simulink model "PIDPositionerF141"  (Simulink 9.1)
settings: Solver=ode4  StartTime=0.0  StopTime=3  RelTol=1e-3  EnableMultiTasking=on
StopFcn:
  | %extract data from structure and plot vs time
  | %Birdsong 10/20/06
  | %This file is copied into the PIDPositioner.mdl Stop callback function
  | %at file/model properites/Callbacks/StopFcn
  | %extract vectors from structure data
  | 
  | %first extract vector data from structure data
  | pid_out=expdata.signals(1).values;
  | des_pos=expdata.signals(2).values(:,1);
  | meas_pos=expdata.signals(2).values(:,2);
  | t=expdata.time;
  | 
  | %plot data in a new figure
  | figure(1);subplot(211)
  | plot(t,pid_out);grid;
  | %axis([0,5,-12,12]);
  | xlabel('Time (sec)');
  | ylabel('PID Controller Ouput (volts)');
  | kp=get_param(strcat(gcs,'/PID Controller'), 'P'); %must match mdl file name exactly
  | ki=get_param(strcat(gcs,'/PID Controller'), 'I');
  | kd=get_param(strcat(gcs,'/PID Controller'), 'D');
  | plot_title=['Closed-Loop PID Controller Sysetm Response Kp=' num2str(kp) ', Ki=' num2str(ki) ', Kd=' num2str(kd)];
  | title(plot_title);
  | 
  | subplot(212);
  | plot(t,des_pos,'--',t,meas_pos,'-');grid;
  | xlabel('Time (sec)');
  | ylabel('Displacement (inches)');
  | legend('desired','measured');
  | %maxlim=1.1*max(max(meas_pos(2000:5000)),max(des_pos(2000:5000)));
  | %minlim=1.1*min(min(meas_pos(2000:5000)),min(des_pos(2000:5000)));
  | %axis([0,5,minlim,maxlim]); %adjust scale account for large offset from any initial drift
values from neighbouring files (symbols this model uses):
  expdata =     [PD10_0.01workspace.mat]    (also in PD42.5_0.1workspace.mat; PID47.5_12_0.15workspace.mat; POnly82workspace.mat; rampP10workspace.mat)
undefined symbols (not defined in the file or in its folder): MIO, National_Instruments, PCI
libraries: sldrtlib x2, simulink_need_slupdate x1, simulink x1
settings Model: Creator=Houska  LastModifiedBy=melab2  SimulationMode=external  ExtModeTrigDuration=10000
settings DataIOCC: LimitDataPoints=on  SignalLoggingSaveFormat=ModelDataLogs  SaveOutput=off  SaveTime=off  SignalLoggingName=logsOut
settings OptimizationCC: ExpressionDepthLimit=2147483647  InitFltsAndDblsToZero=on  LifeSpan=auto
settings DebuggingCC: SaveWithParameterizedLinksMsg=none  SignalResolutionControl=TryResolveAllWithWarning  MultiTaskDSMMsg=warning  MultiTaskCondExecSysMsg=none  FcnCallInpInsideContextMsg=warning  StateNameClashWarn=warning
settings HardwareCC: ProdBitPerPointer=64  ProdBitPerSizeT=64  ProdBitPerPtrDiffT=64  ProdLargestAtomicFloat=Float  ProdIntDivRoundTo=Zero  ProdEndianess=LittleEndian  ProdWordSize=64  ProdHWDeviceType=Intel->x86-64 (Windows64)
settings RTWCC: SystemTargetFile=sldrt.tlc  TemplateMakefile=sldrt.tmf  Description=Simulink Desktop Real-Time  RTWCompilerOptimization=on
settings CodeAppCC: MaxIdLength=95
settings SimulinkDesktopRealTimeCC: TargetPreCompLibLocation=C:\Program Files\MATLAB\R2018a\toolbox\sldrt\lib\win64  TargetLangStandard=C89/C90 (ANSI)  ModelReferenceCompliant=off  CompOptLevelCompliant=off  SupportVariableSizeSignals=off
settings ConfigComp: CovSFcnEnable=off

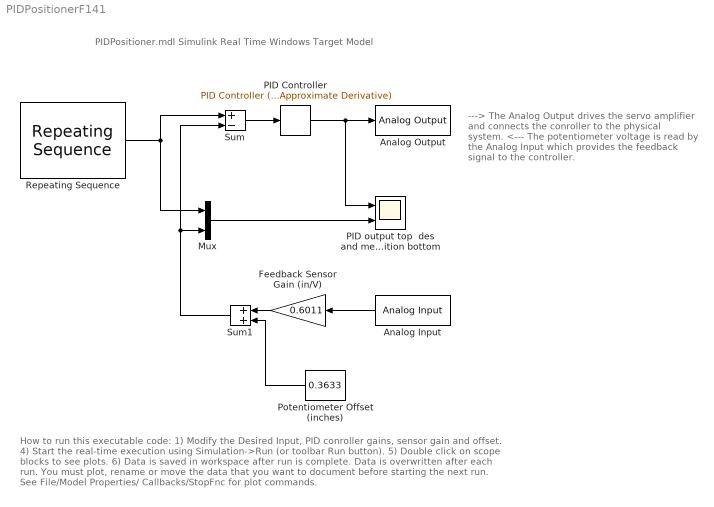
== system PIDPositionerF141 ==
  note: How to run this executable code:
      |
      | 1) Modify the Desired Input, PID conroller gains, sensor gain and offset.
      |
      | 4) Start the real-time execution using Simulation->Run (or toolbar Run button).
      |
      | 5) Double click on scope blocks to see plots.
      |
      | 6) Data is saved in workspace after run is complete.  Data is overwritten after each run.  You must plot,
      | rename or move the data that you want to document before starting the next run.  See File/Model Properties/
      | Callbacks/StopFnc for plot commands.
  note: ---> The Analog Output drives
      | the servo amplifier and
      | connects the conroller to
      | the physical system.
      |
      |
      |
      |
      |
      |
      |
      |
      | <--- The potentiometer voltage
      | is read by the Analog Input
      | which provides the feedback
      | signal to the controller.
  note: PIDPositioner.mdl
      | Simulink Real Time Windows Target Model
  Analog Input : sldrtlib/Analog Input  SampleTime=1e-3  MaxMissedTicks=10  ShowMissedTicks=off  YieldWhenWaiting=off  DrvName=National_Instruments/PCI-MIO-16E-4  DrvAddress=4294967295  DrvOptions=[0 0 0 0 0]  Channels=2  RangeMode=1  VoltRange=1  DataType=1
      settings: AttributesFormatString=National Instruments\nPCI-MIO-16E-4 [auto]  SourceProductName=Simulink Desktop Real-Time
  Analog Output : sldrtlib/Analog Output  SampleTime=1e-3  MaxMissedTicks=10  ShowMissedTicks=off  YieldWhenWaiting=off  DrvName=National_Instruments/PCI-MIO-16E-4  DrvAddress=4294967295  DrvOptions=[0 0 0 0 0]  Channels=1  RangeMode=1  VoltRange=1  InitialValue=0  FinalValue=0
      settings: AttributesFormatString=National Instruments\nPCI-MIO-16E-4 [auto]  SourceProductName=Simulink Desktop Real-Time
  Feedback Sensor Gain (in/V) : Gain  Gain=0.6011
  Mux : Mux  Inputs=2
  PID Controller : simulink_need_slupdate/PID Controller (with Approximate Derivative)  P=82  I=0  D=0  N=600
      settings: SourceProductName=Simulink  SourceProductBaseCode=SL
  PID output top  des and meas position bottom : Scope  NumInputPorts=2
  Potentiometer Offset (inches) : Constant  Value=0.3633
  Repeating Sequence : simulink/Sources/Repeating Sequence  rep_seq_t=[0 1 1.001 1.999 2]  rep_seq_y=[0 0 .2 .2 0]
  Sum : Sum  Inputs=+-  SaturateOnIntegerOverflow=on  InputSameDT=on  OutDataTypeStr=Inherit: Same as first input
  Sum1 : Sum  SaturateOnIntegerOverflow=on  InputSameDT=on  OutDataTypeStr=Inherit: Same as first input
  wires:
  Repeating Sequence/1 -> Sum/1, Mux/1
  PID Controller/1 -> Analog Output/1, PID output top  des and meas position bottom/1
  Sum/1 -> PID Controller/1
  Analog Input/1 -> Feedback Sensor Gain (in/V)/1
  Feedback Sensor Gain (in/V)/1 -> Sum1/1
  Potentiometer Offset (inches)/1 -> Sum1/2
  Sum1/1 -> Sum/2, Mux/2
  Mux/1 -> PID output top  des and meas position bottom/2
